simulink model "ExtendedKalmanFIlterRover"  (R2021a)
settings: Solver=VariableStepAuto  StartTime=0.0  StopTime=60.0  RelTol=1e-3
model workspace (MAT data in the model file):
  Gps_Data = Simulink.Signal
  Gps_Data.DataType = 'auto'
  Gps_Data.Dimensions = -1
  Gps_Data.DimensionsMode = 'auto'
  Gps_Data.Complexity = 'auto'
  Gps_Data.SampleTime = -1
  Gps_Data.SamplingMode = 'auto'
values from neighbouring files (symbols this model uses):
  Kr = 1.0000e-01    (= 0.1)    [parameters.m]
  Q = 1.2e-3    (= 0.0012)    [parameters.m]
  R = 5e-6    (= 5e-06)    [parameters.m]
  Ts = 0.01    [parameters.m]
undefined symbols (not defined in the file or in its folder): K
libraries: robotlib x9, sharedTrackingLibrary x1
settings Model: Creator=user  LastModifiedBy=User
settings SolverCC: AlgebraicLoopSolver=TrustRegion
settings DebuggingCC: SFMachineParentedDataDiag=warning

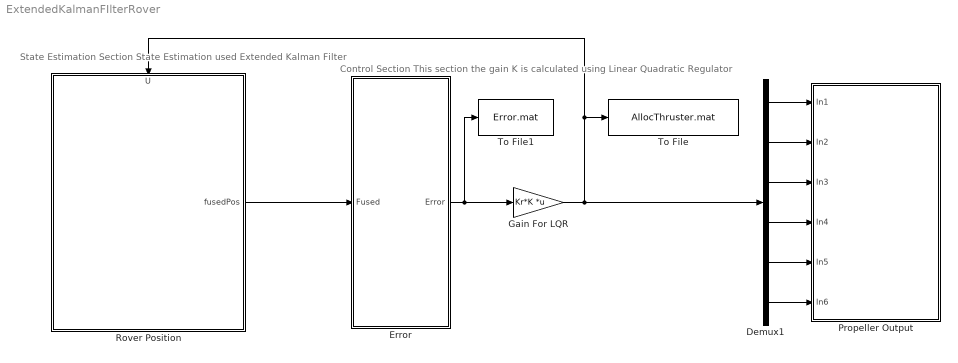
== system ExtendedKalmanFIlterRover ==
  note: State Estimation Section
      |
      | State Estimation used Extended Kalman Filter
  note: Control Section
      |
      | This section the gain K is calculated using Linear Quadratic Regulator
  Demux1 : Demux  Outputs=6
  Error : MATLAB Function  TreatAsAtomicUnit=on
  Gain For LQR : Gain  Gain=Kr*K  Multiplication=Matrix(K*u)  RndMeth=Round
  Propeller Output : Subsystem
  Rover Position : Subsystem
      settings: PortSchema="{\"entries\":[{\"content\":{\"sides\":[{\"content\":{\"connectorIds\":[]},\"type\":\"ConnectorPlacement.EquallySpacedRectSide\",\"uuid\":\"70bf1008-d6b2-49b6-af88-753ab581769c\"},{\"content\":{\"connectorIds\":[\"Out1\"],\"side\":\"RIGHT\"},\"type\":\"ConnectorPlacement.EquallySpacedRectSide\",\"uuid\":\"04ddecda-8c46-4437-987b-fe54c22cd984\"},{\"content\":{\"connectorIds\":[\"In1\"],\"side\":\"TOP\"},\"type\":\"ConnectorPlacement.EquallySpacedRectSide\",\"uuid\":\"625a0b2a-12f2-4858-86ad-539843868268\"}]},\"type\":\"ConnectorPlacement.EquallySpacedConnector\",\"uuid\":\"e8b3dc5a-c0d9-4ca2-a6c5-b2c7be1821de\"}],\"packageUris\":[\"http://schema.mathworks.com/mf0/Connector/R2020b\"],\"version\":\"1.0\"}"
  To File : ToFile  Filename=AllocThruster.mat  SaveFormat=Timeseries  SampleTime=Ts
  To File1 : ToFile  Filename=Error.mat  MatrixName=Error  SaveFormat=Timeseries  SampleTime=Ts
  wires:
  Demux1/1 -> Propeller Output/1(In1)
  Demux1/2 -> Propeller Output/2(In2)
  Demux1/3 -> Propeller Output/3(In3)
  Demux1/4 -> Propeller Output/4(In4)
  Demux1/5 -> Propeller Output/5(In5)
  Demux1/6 -> Propeller Output/6(In6)
  Error/1(Error) -> Gain For LQR/1, To File1/1
  Rover Position/1(fusedPos) -> Error/1(Fused)
  Gain For LQR/1 -> Demux1/1, To File/1, Rover Position/1(U)

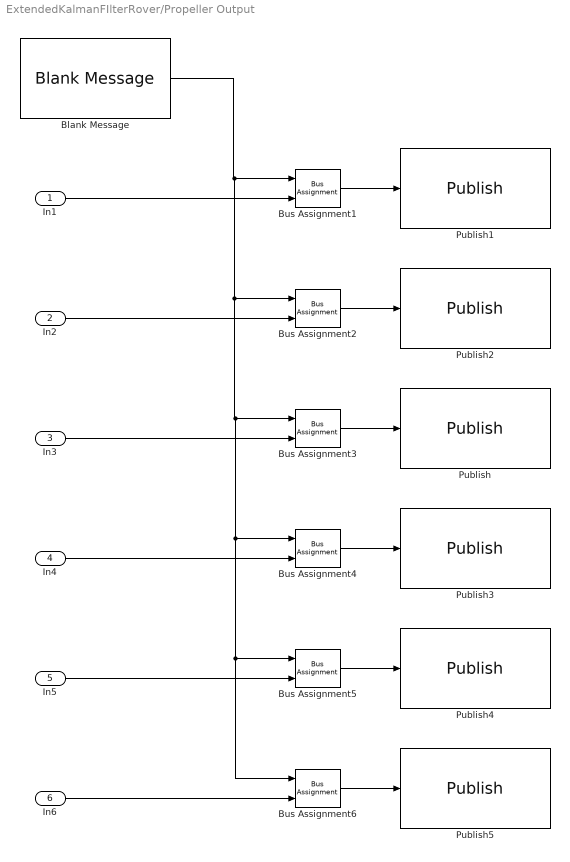
== system ExtendedKalmanFIlterRover/Propeller Output ==
  In1 : Inport
  In2 : Inport  Port=2
  In3 : Inport  Port=3
  In4 : Inport  Port=4
  In5 : Inport  Port=5
  In6 : Inport  Port=6
  Blank Message : robotlib/Blank Message  messageClass=Message  entityType=uuv_gazebo_ros_plugins_msgs/FloatStamped  messageType=uuv_gazebo_ros_plugins_msgs/FloatStamped  SampleTime=inf  legacyBusStruct=off
  Bus Assignment{1..6} (6 alike) : BusAssignment  AssignedSignals=Data
  Publish : robotlib/Publish  topicSource=Select from ROS network  topic=/bluerov2/thrusters/2/input  messageType=uuv_gazebo_ros_plugins_msgs/FloatStamped  legacyBusStruct=off  messageQueueLength=1
  Publish1 : robotlib/Publish  topicSource=Select from ROS network  topic=/bluerov2/thrusters/0/input  messageType=uuv_gazebo_ros_plugins_msgs/FloatStamped  legacyBusStruct=off  messageQueueLength=1
  Publish2 : robotlib/Publish  topicSource=Select from ROS network  topic=/bluerov2/thrusters/1/input  messageType=uuv_gazebo_ros_plugins_msgs/FloatStamped  legacyBusStruct=off  messageQueueLength=1
  Publish3 : robotlib/Publish  topicSource=Select from ROS network  topic=/bluerov2/thrusters/3/input  messageType=uuv_gazebo_ros_plugins_msgs/FloatStamped  legacyBusStruct=off  messageQueueLength=1
  Publish4 : robotlib/Publish  topicSource=Select from ROS network  topic=/bluerov2/thrusters/4/input  messageType=uuv_gazebo_ros_plugins_msgs/FloatStamped  legacyBusStruct=off  messageQueueLength=1
  Publish5 : robotlib/Publish  topicSource=Select from ROS network  topic=/bluerov2/thrusters/5/input  messageType=uuv_gazebo_ros_plugins_msgs/FloatStamped  legacyBusStruct=off  messageQueueLength=1
  wires:
  Bus Assignment5/1 -> Publish4/1
  Bus Assignment4/1 -> Publish3/1
  Bus Assignment3/1 -> Publish/1
  Bus Assignment2/1 -> Publish2/1
  Bus Assignment1/1 -> Publish1/1
  Bus Assignment6/1 -> Publish5/1
  Blank Message/1 -> Bus Assignment6/1, Bus Assignment5/1, Bus Assignment4/1, Bus Assignment3/1, Bus Assignment2/1, Bus Assignment1/1
  In1/1 -> Bus Assignment1/2
  In2/1 -> Bus Assignment2/2
  In3/1 -> Bus Assignment3/2
  In4/1 -> Bus Assignment4/2
  In5/1 -> Bus Assignment5/2
  In6/1 -> Bus Assignment6/2

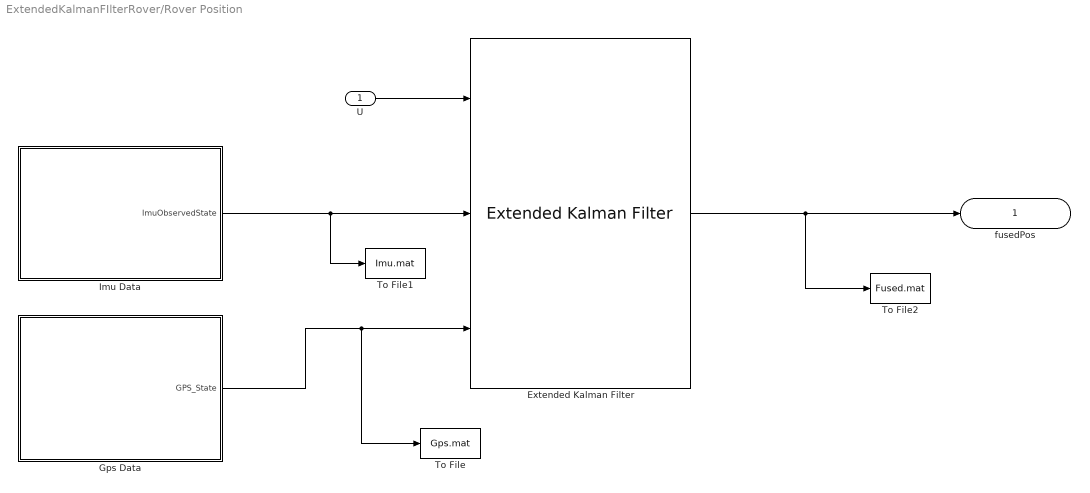
== system ExtendedKalmanFIlterRover/Rover Position ==
  U : Inport
  Extended Kalman Filter : sharedTrackingLibrary/Extended Kalman Filter  StateTransitionFcn=myStateTransitionFcn  HasStateTransitionJacobianFcn=off  HasAdditiveProcessNoise=Additive  ProcessNoise=diag([Q Q Q Q Q Q Q Q Q Q Q Q])  HasTimeVaryingProcessNoise=off  HasStateTransitionFcnExtraArgument=1  InitialState=[0 0 0 0 0 0 0 0 0 0 0 0]  InitialStateCovariance=1e-5  MeasurementFcn1=ImuMeasurementFcn  HasMeasurementJacobianFcn1=off  HasMeasurementEnablePort1=off  HasAdditiveMeasurementNoise1=Additive  MeasurementNoise1=diag([R R R R R R])  HasTimeVaryingMeasurementNoise1=off  HasMeasurementFcnExtraArgument1=0  MeasurementFcn2=GpsMeasurementFcn  HasMeasurementJacobianFcn2=off  HasMeasurementEnablePort2=off  HasAdditiveMeasurementNoise2=Additive  MeasurementNoise2=diag([R R R])  HasTimeVaryingMeasurementNoise2=off  HasMeasurementFcnExtraArgument2=0  MeasurementFcn3=myMeasurementFcn  HasMeasurementJacobianFcn3=off  HasMeasurementEnablePort3=off  HasAdditiveMeasurementNoise3=Additive  MeasurementNoise3=1  HasTimeVaryingMeasurementNoise3=off  HasMeasurementFcnExtraArgument3=0  MeasurementFcn4=myMeasurementFcn  HasMeasurementJacobianFcn4=off  HasMeasurementEnablePort4=off  HasAdditiveMeasurementNoise4=Additive  MeasurementNoise4=1  HasTimeVaryingMeasurementNoise4=off  HasMeasurementFcnExtraArgument4=0  MeasurementFcn5=myMeasurementFcn  HasMeasurementJacobianFcn5=off  HasMeasurementEnablePort5=off  HasAdditiveMeasurementNoise5=Additive  MeasurementNoise5=1  HasTimeVaryingMeasurementNoise5=off  HasMeasurementFcnExtraArgument5=0  EnableMultirate=off  StateTransitionFcnSampleTime=1  MeasurementFcn1SampleTime=1  MeasurementFcn2SampleTime=1  MeasurementFcn3SampleTime=1  MeasurementFcn4SampleTime=1  MeasurementFcn5SampleTime=1  UseCurrentEstimator=on  OutputStateCovariance=off  DataType=double  SampleTime=Ts  NumberOfMeasurements=2
      settings: SourceProductBaseCode=CT,DR,TF,ID,LP,NV,AR,RO,RR,UV,VE
  Gps Data : Subsystem
  Imu Data : Subsystem
  To File : ToFile  Filename=Gps.mat  MatrixName=Coordinate  SaveFormat=Timeseries  SampleTime=Ts
  To File1 : ToFile  Filename=Imu.mat  MatrixName=ImuCoordinate  SaveFormat=Timeseries  SampleTime=Ts
  To File2 : ToFile  Filename=Fused.mat  MatrixName=Fused  SaveFormat=Timeseries  SampleTime=Ts
  fusedPos : Outport
  wires:
  Extended Kalman Filter/1 -> To File2/1, fusedPos/1
  Imu Data/1(ImuObservedState) -> To File1/1, Extended Kalman Filter/2
  U/1 -> Extended Kalman Filter/1
  Gps Data/1(GPS_State) -> To File/1, Extended Kalman Filter/3

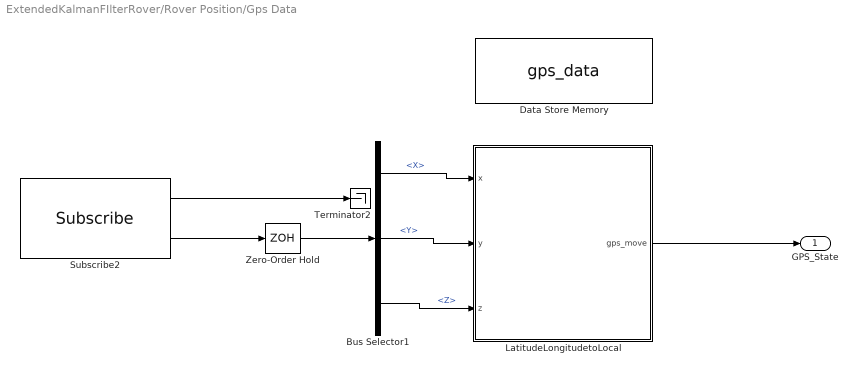
== system ExtendedKalmanFIlterRover/Rover Position/Gps Data ==
  Bus Selector1 : BusSelector  OutputSignals=Pose.Pose.Position.X,Pose.Pose.Position.Y,Pose.Pose.Position.Z
  Data Store Memory : DataStoreMemory  DataStoreName=gps_data  ReadBeforeWriteMsg=warning  WriteAfterWriteMsg=warning  WriteAfterReadMsg=warning  InitialValue=[0;0;0]  VectorParams1D=off  ShowAdditionalParam=off  OutDataTypeStr=double
  LatitudeLongitudetoLocal : MATLAB Function  TreatAsAtomicUnit=on  SystemSampleTime=Ts
  Subscribe2 : robotlib/Subscribe  topicSource=Select from ROS network  topic=/gps_conv  messageType=nav_msgs/Odometry  SampleTime=-1  legacyBusStruct=off  messageQueueLength=1
  Terminator2 : Terminator
  Zero-Order Hold : ZeroOrderHold  SampleTime=Ts
  GPS_State : Outport
  wires:
  LatitudeLongitudetoLocal/1(gps_move) -> GPS_State/1
  Subscribe2/1 -> Terminator2/1
  Bus Selector1/1 -> LatitudeLongitudetoLocal/1(x)  "<X>"
  Bus Selector1/3 -> LatitudeLongitudetoLocal/3(z)  "<Z>"
  Bus Selector1/2 -> LatitudeLongitudetoLocal/2(y)  "<Y>"
  Zero-Order Hold/1 -> Bus Selector1/1
  Subscribe2/2 -> Zero-Order Hold/1

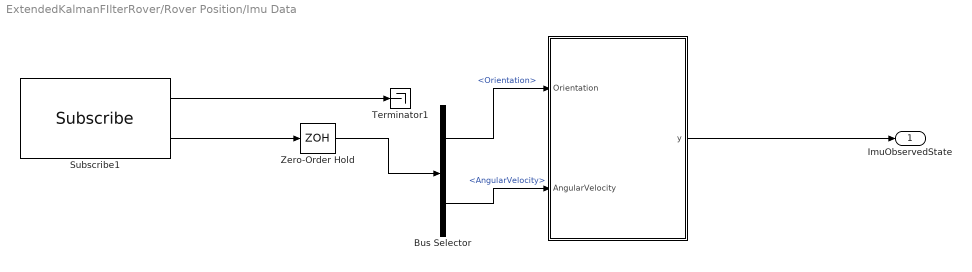
== system ExtendedKalmanFIlterRover/Rover Position/Imu Data ==
  " " : MATLAB Function  TreatAsAtomicUnit=on
  Bus Selector : BusSelector  OutputSignals=Orientation,AngularVelocity
  Subscribe1 : robotlib/Subscribe  topicSource=Select from ROS network  topic=/bluerov2/imu  messageType=sensor_msgs/Imu  SampleTime=-1  legacyBusStruct=off  messageQueueLength=1
  Terminator1 : Terminator
  Zero-Order Hold : ZeroOrderHold  SampleTime=Ts
  ImuObservedState : Outport
  wires:
  Subscribe1/1 -> Terminator1/1
  " "/1(y) -> ImuObservedState/1
  Zero-Order Hold/1 -> Bus Selector/1
  Subscribe1/2 -> Zero-Order Hold/1
  Bus Selector/1 -> " "/1(Orientation)  "<Orientation>"
  Bus Selector/2 -> " "/2(AngularVelocity)  "<AngularVelocity>"

== matlab function ExtendedKalmanFIlterRover/Rover Position/Gps Data/LatitudeLongitudetoLocal ==
  data: x input; gps_move output; y input; z input; gps_data data_store_memory
function gps_move = fcn(x,y,z)
global gps_data;

gps_data(1) = x - 468441.325499; 
gps_data(2) = y - 3713776.85777;
gps_data(3) = z ;

gps_move = gps_data;

== matlab function ExtendedKalmanFIlterRover/Error ==
  data: Fused input; Error output
function Error = fcn(Fused)

%Set your reference
reference = [100;0;0;0;0;0;0;0;0;0;0;0];
Error = reference-Fused;

== matlab function ExtendedKalmanFIlterRover/Rover Position/Imu Data/  ==
  data: Orientation input; y output; AngularVelocity input
function y = fcn(Orientation,AngularVelocity)




y = [Orientation.X;Orientation.Y;Orientation.Z;AngularVelocity.X;AngularVelocity.Y;AngularVelocity.Z];
